simulink model "stage_02"  (R2021b)
settings: Solver=daessc  StartTime=0.0  StopTime=2500  FixedStep=0.001  RelTol=1e-3
values from neighbouring files (symbols this model uses):
  Inom_FC1 = 50    [initParams.m]
  Inom_FC2 = 50    [initParams.m]
  Pnom_FC = 25000    [initParams.m]
  Vnom = 500    [initParams.m]
undefined symbols (not defined in the file or in its folder): Bat, DiscIntNeverNeededParam, Mot
libraries: fl_lib x21, nesl_utility x14, ee_lib x4
settings Model: Creator=gdudgeon  LastModifiedBy=gdudgeon

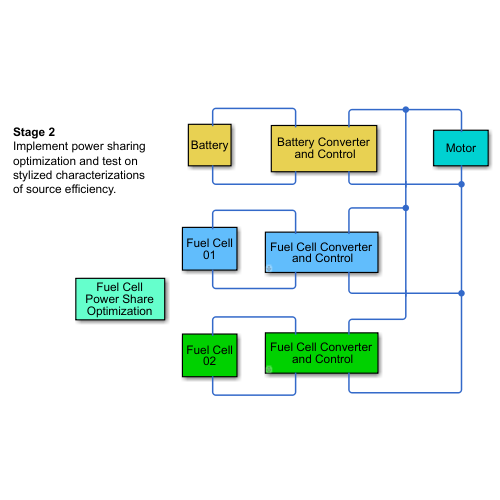
[thumbnail: Simulink's stored preview of the top-level diagram]
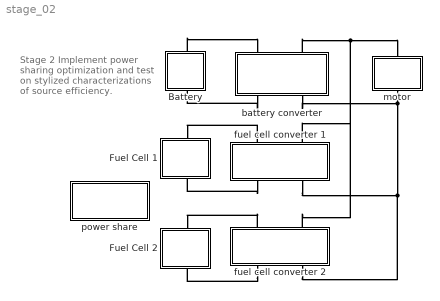
== system stage_02 ==
  note: Stage 2
      | Implement power sharing optimization and test on stylized characterizations of source efficiency.
  Battery : Subsystem
      settings: PortSchema="{\"entries\":[{\"content\":{\"sides\":[{\"content\":{\"connectorIds\":[]},\"type\":\"ConnectorPlacement.EquallySpacedRectSide\",\"uuid\":\"a686e7db-b3c2-4e82-90e1-b07be3e28f3a\"},{\"content\":{\"connectorIds\":[],\"side\":\"RIGHT\"},\"type\":\"ConnectorPlacement.EquallySpacedRectSide\",\"uuid\":\"0e51eb8c-8945-4106-9b2f-04139f0293aa\"},{\"content\":{\"connectorIds\":[\"LConn1\"],\"side\":\"TOP\"},\"type\":\"ConnectorPlacement.EquallySpacedRectSide\",\"uuid\":\"6b60bb75-cfc3-4157-9141-8615eb9e37cb\"},{\"content\":{\"connectorIds\":[\"RConn1\"],\"side\":\"BOTTOM\"},\"type\":\"ConnectorPlacement.EquallySpacedRectSide\",\"uuid\":\"c1a51cb3-7790-499e-bd85-73216263d646\"}]},\"type\":\"ConnectorPlacement.EquallySpacedConnector\",\"uuid\":\"ef7b4de5-6239-4f21-bedd-9a9241ffad20\"}],\"packageUris\":[\"http://schema.mathworks.com/mf0/Connector/R2020b\"],\"version\":\"1.0\"}"
      mask Display: disp('Battery')
  Fuel Cell 1 : Subsystem
      settings: PortSchema="{\"entries\":[{\"content\":{\"sides\":[{\"content\":{\"connectorIds\":[]},\"type\":\"ConnectorPlacement.EquallySpacedRectSide\",\"uuid\":\"a686e7db-b3c2-4e82-90e1-b07be3e28f3a\"},{\"content\":{\"connectorIds\":[],\"side\":\"RIGHT\"},\"type\":\"ConnectorPlacement.EquallySpacedRectSide\",\"uuid\":\"0e51eb8c-8945-4106-9b2f-04139f0293aa\"},{\"content\":{\"connectorIds\":[\"LConn1\"],\"side\":\"TOP\"},\"type\":\"ConnectorPlacement.EquallySpacedRectSide\",\"uuid\":\"6b60bb75-cfc3-4157-9141-8615eb9e37cb\"},{\"content\":{\"connectorIds\":[\"RConn1\"],\"side\":\"BOTTOM\"},\"type\":\"ConnectorPlacement.EquallySpacedRectSide\",\"uuid\":\"6246c242-d76b-4057-8f90-ef1191bb40d6\"}]},\"type\":\"ConnectorPlacement.EquallySpacedConnector\",\"uuid\":\"ef7b4de5-6239-4f21-bedd-9a9241ffad20\"}],\"packageUris\":[\"http://schema.mathworks.com/mf0/Connector/R2020b\"],\"version\":\"1.0\"}"
      mask Display: disp('Fuel Cell\n01')
  Fuel Cell 2 : Subsystem
      settings: PortSchema="{\"entries\":[{\"content\":{\"sides\":[{\"content\":{\"connectorIds\":[]},\"type\":\"ConnectorPlacement.EquallySpacedRectSide\",\"uuid\":\"a686e7db-b3c2-4e82-90e1-b07be3e28f3a\"},{\"content\":{\"connectorIds\":[],\"side\":\"RIGHT\"},\"type\":\"ConnectorPlacement.EquallySpacedRectSide\",\"uuid\":\"0e51eb8c-8945-4106-9b2f-04139f0293aa\"},{\"content\":{\"connectorIds\":[\"LConn1\"],\"side\":\"TOP\"},\"type\":\"ConnectorPlacement.EquallySpacedRectSide\",\"uuid\":\"6b60bb75-cfc3-4157-9141-8615eb9e37cb\"},{\"content\":{\"connectorIds\":[\"RConn1\"],\"side\":\"BOTTOM\"},\"type\":\"ConnectorPlacement.EquallySpacedRectSide\",\"uuid\":\"6246c242-d76b-4057-8f90-ef1191bb40d6\"}]},\"type\":\"ConnectorPlacement.EquallySpacedConnector\",\"uuid\":\"ef7b4de5-6239-4f21-bedd-9a9241ffad20\"}],\"packageUris\":[\"http://schema.mathworks.com/mf0/Connector/R2020b\"],\"version\":\"1.0\"}"
      mask Display: disp('Fuel Cell\n02')
  battery converter : Subsystem
      settings: PortSchema="{\"entries\":[{\"content\":{\"sides\":[{\"content\":{\"connectorIds\":[]},\"type\":\"ConnectorPlacement.EquallySpacedRectSide\",\"uuid\":\"465408c9-80bd-457c-883a-4a132321254b\"},{\"content\":{\"connectorIds\":[],\"side\":\"RIGHT\"},\"type\":\"ConnectorPlacement.EquallySpacedRectSide\",\"uuid\":\"04120ebf-e4ec-443f-a627-4e992580e56f\"},{\"content\":{\"connectorIds\":[\"LConn1\",\"LConn2\"],\"side\":\"TOP\"},\"type\":\"ConnectorPlacement.EquallySpacedRectSide\",\"uuid\":\"0ef2b150-f732-4ac6-bc9b-74fd7e496e19\"},{\"content\":{\"connectorIds\":[\"RConn1\",\"RConn2\"],\"side\":\"BOTTOM\"},\"type\":\"ConnectorPlacement.EquallySpacedRectSide\",\"uuid\":\"3ceaa64c-40e0-49b8-9128-82da92f184b4\"}]},\"type\":\"ConnectorPlacement.EquallySpacedConnector\",\"uuid\":\"70c8e7cc-610c-4e7a-9707-57af70b2f144\"}],\"packageUris\":[\"http://schema.mathworks.com/mf0/Connector/R2020b\"],\"version\":\"1.0\"}"
      mask Display: disp('Battery Converter\n and Control')
  fuel cell converter 1 : Subsystem  mask{Vref=Vnom, Imax=Inom_FC1}
      mask prompts: Vref "Voltage Setpoint (V)"; Imax "Maximum Current (A)"
      settings: PortSchema="{\"entries\":[{\"content\":{\"sides\":[{\"content\":{\"connectorIds\":[]},\"type\":\"ConnectorPlacement.EquallySpacedRectSide\",\"uuid\":\"465408c9-80bd-457c-883a-4a132321254b\"},{\"content\":{\"connectorIds\":[],\"side\":\"RIGHT\"},\"type\":\"ConnectorPlacement.EquallySpacedRectSide\",\"uuid\":\"04120ebf-e4ec-443f-a627-4e992580e56f\"},{\"content\":{\"connectorIds\":[\"LConn1\",\"LConn2\"],\"side\":\"TOP\"},\"type\":\"ConnectorPlacement.EquallySpacedRectSide\",\"uuid\":\"0ef2b150-f732-4ac6-bc9b-74fd7e496e19\"},{\"content\":{\"connectorIds\":[\"RConn1\",\"RConn2\"],\"side\":\"BOTTOM\"},\"type\":\"ConnectorPlacement.EquallySpacedRectSide\",\"uuid\":\"cccf9d02-f6c7-4a15-ab4f-a4dd83d7ce46\"}]},\"type\":\"ConnectorPlacement.EquallySpacedConnector\",\"uuid\":\"70c8e7cc-610c-4e7a-9707-57af70b2f144\"}],\"packageUris\":[\"http://schema.mathworks.com/mf0/Connector/R2020b\"],\"version\":\"1.0\"}"
      mask Display: disp('Fuel Cell Converter\n and Control')
  fuel cell converter 2 : Subsystem  mask{Vref=Vnom, Imax=Inom_FC2}
      mask prompts: Vref "Voltage Setpoint (V)"; Imax "Maximum Current (A)"
      settings: PortSchema="{\"entries\":[{\"content\":{\"sides\":[{\"content\":{\"connectorIds\":[]},\"type\":\"ConnectorPlacement.EquallySpacedRectSide\",\"uuid\":\"465408c9-80bd-457c-883a-4a132321254b\"},{\"content\":{\"connectorIds\":[],\"side\":\"RIGHT\"},\"type\":\"ConnectorPlacement.EquallySpacedRectSide\",\"uuid\":\"04120ebf-e4ec-443f-a627-4e992580e56f\"},{\"content\":{\"connectorIds\":[\"LConn1\",\"LConn2\"],\"side\":\"TOP\"},\"type\":\"ConnectorPlacement.EquallySpacedRectSide\",\"uuid\":\"0ef2b150-f732-4ac6-bc9b-74fd7e496e19\"},{\"content\":{\"connectorIds\":[\"RConn1\",\"RConn2\"],\"side\":\"BOTTOM\"},\"type\":\"ConnectorPlacement.EquallySpacedRectSide\",\"uuid\":\"cccf9d02-f6c7-4a15-ab4f-a4dd83d7ce46\"}]},\"type\":\"ConnectorPlacement.EquallySpacedConnector\",\"uuid\":\"70c8e7cc-610c-4e7a-9707-57af70b2f144\"}],\"packageUris\":[\"http://schema.mathworks.com/mf0/Connector/R2020b\"],\"version\":\"1.0\"}"
      mask Display: disp('Fuel Cell Converter\n and Control')
  motor : Subsystem
      mask Display: disp('Motor')
  power share : Subsystem
      mask Display: disp('Fuel Cell\nPower Share\nOptimization')
  connections:
  motor/RConn1 -- battery converter/RConn2 -- fuel cell converter 2/RConn2 -- fuel cell converter 1/RConn2
  battery converter/LConn2 -- motor/LConn1 -- fuel cell converter 2/LConn2 -- fuel cell converter 1/LConn2
  fuel cell converter 1/LConn1 -- Fuel Cell 1/LConn1
  fuel cell converter 1/RConn1 -- Fuel Cell 1/RConn1
  Battery/LConn1 -- battery converter/LConn1
  battery converter/RConn1 -- Battery/RConn1
  fuel cell converter 2/RConn1 -- Fuel Cell 2/RConn1
  fuel cell converter 2/LConn1 -- Fuel Cell 2/LConn1

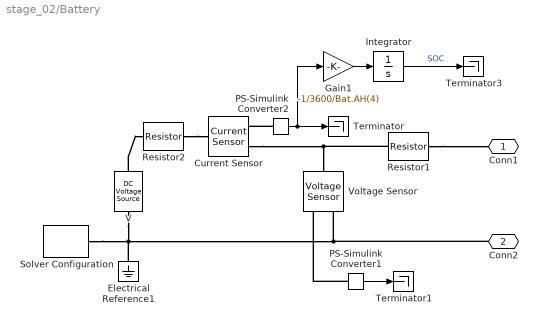
== system stage_02/Battery ==
  Current Sensor : fl_lib/Electrical/Electrical Sensors/Current Sensor
  Electrical Reference1 : fl_lib/Electrical/Electrical Elements/Electrical Reference
  Gain1 : Gain  Gain=-1/3600/Bat.AH(4)
  Integrator : Integrator  InitialCondition=Bat.initSOC
  PS-Simulink Converter1 : nesl_utility/PS-Simulink Converter  PhysicalDomain=network_engine_domain  SubClassName=ps_output  LeftPortType=input  RightPortType=output  PseudoPeriodic=off  Frequencies=[]  Unit=inherit  AffineConversion=off
      settings: SourceProductBaseCode=PW,SS
  PS-Simulink Converter2 : nesl_utility/PS-Simulink Converter  PhysicalDomain=network_engine_domain  SubClassName=ps_output  LeftPortType=input  RightPortType=output  PseudoPeriodic=off  Frequencies=[]  Unit=inherit  AffineConversion=off
      settings: SourceProductBaseCode=PW,SS
  Resistor1 : fl_lib/Electrical/Electrical Elements/Resistor  R=1e-3 Ohm  i_specify=off  i_priority=None  i=0 A  i_nominal_specify=off  i_nominal_unit=A  i_nominal_value=1  v_specify=off  v_priority=None  v=0 V  v_nominal_specify=off  v_nominal_unit=V  v_nominal_value=1
  Resistor2 : fl_lib/Electrical/Electrical Elements/Resistor  R=Bat.R0(4,4) Ohm  i_specify=off  i_priority=None  i=0 A  i_nominal_specify=off  i_nominal_unit=A  i_nominal_value=1  v_specify=off  v_priority=None  v=0 V  v_nominal_specify=off  v_nominal_unit=V  v_nominal_value=1
  Solver Configuration : nesl_utility/Solver Configuration  PhysicalDomain=network_engine_domain  SubClassName=solver  LeftPortType=input  RightPortType=generic  Tones=[]  Harmonics=[]  SimulateNoise=off  Profile=off  UseLocalSampling=off  EnableSwitchedLinearOptims=on  FrequencyDomain=off  UseCCode=off  RelTol=0.001  AbsTol=1e-06  MinStep=1e-09  ToWorkspace=off  RevertToSquareIcSolve=off  NumHomotopyIterations=100  PhasorMode=off  PhasorModeNumHarmonics=1  DoDC=off  ResidualTolerance=1e-09  UseLocalSolver=off  LocalSolverChoice=NE_BACKWARD_EULER_ADVANCER  LocalSolverSampleTime=0.001  DoFixedCost=off  MaxNonlinIter=3  MaxModeIter=2  ComputeImpulses=off  ImpulseIterations=2  LinearAlgebra=auto  EquationFormulation=NE_TIME_EF  DelaysMemoryBudget=1024  AutomaticFiltering=on  FilteringTimeConstant=0.001  PartitionStorageMethod=AS_NEEDED  PartitionMemoryBudget=1024  PartitionMethod=ROBUST
      settings: SourceProductBaseCode=PW,SS
  Terminator : Terminator
  Terminator1 : Terminator
  Terminator3 : Terminator
  V : fl_lib/Electrical/Electrical Sources/DC Voltage Source  v0=Bat.noLoadV(4,4) V
  Voltage Sensor : fl_lib/Electrical/Electrical Sensors/Voltage Sensor
  Conn1 : PMIOPort  Side=Left
  Conn2 : PMIOPort  Port=2  Side=Right
  wires:
  PS-Simulink Converter2/1 -> Gain1/1, Terminator/1
  PS-Simulink Converter1/1 -> Terminator1/1
  Integrator/1 -> Terminator3/1  "SOC"
  Gain1/1 -> Integrator/1
  connections:
  PS-Simulink Converter2/LConn1 -- Current Sensor/RConn1
  Electrical Reference1/LConn1 -- V/RConn1 -- Solver Configuration/RConn1 -- Conn2/RConn1 -- Voltage Sensor/RConn2
  Current Sensor/RConn2 -- Resistor1/LConn1 -- Voltage Sensor/LConn1
  PS-Simulink Converter1/LConn1 -- Voltage Sensor/RConn1
  Resistor1/RConn1 -- Conn1/RConn1
  V/LConn1 -- Resistor2/LConn1
  Resistor2/RConn1 -- Current Sensor/LConn1

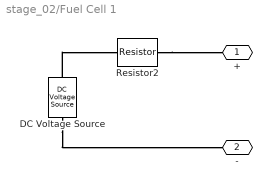
== system stage_02/Fuel Cell 1 ==
  DC Voltage Source : fl_lib/Electrical/Electrical Sources/DC Voltage Source  v0=250 V
  Resistor2 : fl_lib/Electrical/Electrical Elements/Resistor  R=1e-3 Ohm  i_specify=off  i_priority=None  i=0 A  i_nominal_specify=off  i_nominal_unit=A  i_nominal_value=1  v_specify=off  v_priority=None  v=0 V  v_nominal_specify=off  v_nominal_unit=V  v_nominal_value=1
  + : PMIOPort  Side=Left
  - : PMIOPort  Port=2  Side=Right
  connections:
  DC Voltage Source/LConn1 -- Resistor2/LConn1
  Resistor2/RConn1 -- +/RConn1
  DC Voltage Source/RConn1 -- -/RConn1

== system stage_02/Fuel Cell 2 ==
  DC Voltage Source : fl_lib/Electrical/Electrical Sources/DC Voltage Source  v0=250 V
  Resistor2 : fl_lib/Electrical/Electrical Elements/Resistor  R=1e-3 Ohm  i_specify=off  i_priority=None  i=0 A  i_nominal_specify=off  i_nominal_unit=A  i_nominal_value=1  v_specify=off  v_priority=None  v=0 V  v_nominal_specify=off  v_nominal_unit=V  v_nominal_value=1
  + : PMIOPort  Side=Left
  - : PMIOPort  Port=2  Side=Right
  connections:
  DC Voltage Source/RConn1 -- -/RConn1
  Resistor2/RConn1 -- +/RConn1
  DC Voltage Source/LConn1 -- Resistor2/LConn1

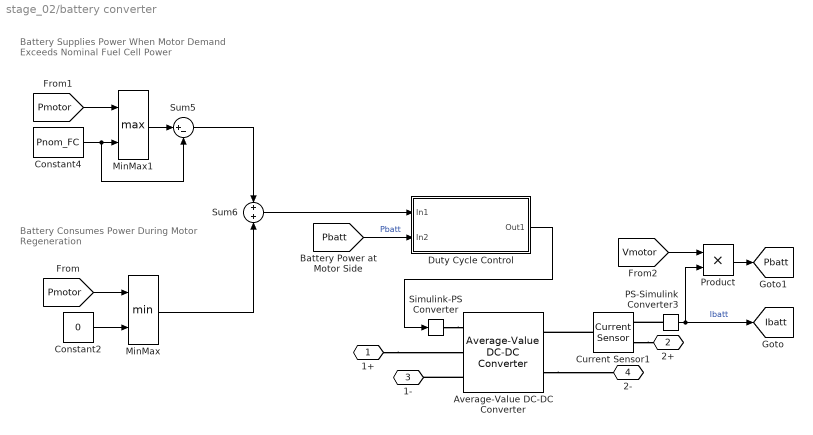
== system stage_02/battery converter ==
  note: Battery Consumes Power
      | During Motor Regeneration
  note: Battery Supplies Power When
      | Motor Demand Exceeds Nominal
      | Fuel Cell Power
  Average-Value DC-DC Converter : ee_lib/Semiconductors & Converters/Converters/Average-Value DC-DC Converter  control_option=ee.enum.converters.controlinput.dutycycle  converter_type=ee.enum.converters.dcdctype.buckboost  efficiency_option=ee.enum.converters.efficiency.constant  efficiency_fixed=100  i_vec=[0, 2, 5] A  efficiency_vec=[90, 95, 98]
      settings: SourceProductBaseCode=PS  InternalSimscapePortConfiguration="{\"Bottom\":[],\"Left\":[{\"id\":\"DutyCycle\",\"label\":\"DutyCycle\",\"type\":\"input\"},{\"id\":\"p1\",\"label\":\"1+\",\"type\":\"foundation.electrical.electrical\"},{\"id\":\"n1\",\"label\":\"1-\",\"type\":\"foundation.electrical.electrical\"}],\"Right\":[{\"id\":\"p2\",\"label\":\"2+\",\"type\":\"foundation.electrical.electrical\"},{\"id\":\"n2\",\"label\":\"2-\",\"type\":\"foundation.electrical.electrical\"}],\"Top\":[]}"
  Constant2 : Constant  Value=0
  Constant4 : Constant  Value=Pnom_FC
  Current Sensor1 : fl_lib/Electrical/Electrical Sensors/Current Sensor
  Duty Cycle Control : Subsystem
      mask Display: disp('Duty-Cycle Control')
  MinMax : MinMax  Inputs=2
  MinMax1 : MinMax  Function=max  Inputs=2
  PS-Simulink Converter3 : nesl_utility/PS-Simulink Converter  PhysicalDomain=network_engine_domain  SubClassName=ps_output  LeftPortType=input  RightPortType=output  PseudoPeriodic=off  Frequencies=[]  Unit=inherit  AffineConversion=off
      settings: SourceProductBaseCode=PW,SS
  Product : Product
  Simulink-PS Converter : nesl_utility/Simulink-PS Converter  PhysicalDomain=network_engine_domain  SubClassName=ps_input  LeftPortType=input  RightPortType=output  PseudoPeriodic=off  Frequencies=[]  NoiseDistribution=none  NoiseParameters=[]  Unit=1  AffineConversion=off  FilteringAndDerivatives=provide  SimscapeFilterOrder=1  InputFilterTimeConstant=0.001  UdotUserProvided=0
      settings: SourceProductBaseCode=PW,SS
  Sum5 : Sum  Inputs=|+-
  Sum6 : Sum
  1+ : PMIOPort  Side=Left
  2+ : PMIOPort  Port=2  Side=Left
  1- : PMIOPort  Port=3  Side=Right
  2- : PMIOPort  Port=4  Side=Right
  tag scope: Ibatt=global, Pbatt=global
  wires:
  Constant4/1 -> Sum5/2, MinMax1/2
  Sum5/1 -> Sum6/1
  MinMax/1 -> Sum6/2
  [Pmotor] -> MinMax1/1
  MinMax1/1 -> Sum5/1
  Constant2/1 -> MinMax/2
  [Pmotor] -> MinMax/1
  PS-Simulink Converter3/1 -> [Ibatt], Product/2  "Ibatt"
  [Pbatt] -> Duty Cycle Control/2(In2)  "Pbatt"
  Duty Cycle Control/1(Out1) -> Simulink-PS Converter/1
  Sum6/1 -> Duty Cycle Control/1(In1)
  [Vmotor] -> Product/1
  Product/1 -> [Pbatt]
  connections:
  PS-Simulink Converter3/LConn1 -- Current Sensor1/RConn1
  Average-Value DC-DC Converter/RConn2 -- 2-/RConn1
  Current Sensor1/LConn1 -- Average-Value DC-DC Converter/RConn1
  Average-Value DC-DC Converter/LConn3 -- 1-/RConn1
  1+/RConn1 -- Average-Value DC-DC Converter/LConn2
  Simulink-PS Converter/RConn1 -- Average-Value DC-DC Converter/LConn1
  Current Sensor1/RConn2 -- 2+/RConn1

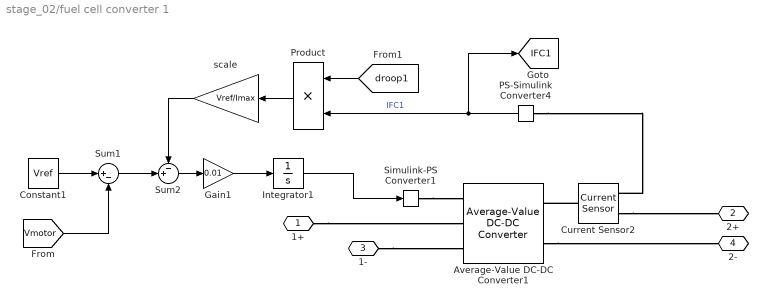
== system stage_02/fuel cell converter 1 ==
  Average-Value DC-DC Converter1 : ee_lib/Semiconductors & Converters/Converters/Average-Value DC-DC Converter  control_option=ee.enum.converters.controlinput.dutycycle  converter_type=ee.enum.converters.dcdctype.buckboost  efficiency_option=ee.enum.converters.efficiency.constant  efficiency_fixed=100  i_vec=[0, 2, 5] A  efficiency_vec=[90, 95, 98]
      settings: SourceProductBaseCode=PS  InternalSimscapePortConfiguration="{\"Bottom\":[],\"Left\":[{\"id\":\"DutyCycle\",\"label\":\"DutyCycle\",\"type\":\"input\"},{\"id\":\"p1\",\"label\":\"1+\",\"type\":\"foundation.electrical.electrical\"},{\"id\":\"n1\",\"label\":\"1-\",\"type\":\"foundation.electrical.electrical\"}],\"Right\":[{\"id\":\"p2\",\"label\":\"2+\",\"type\":\"foundation.electrical.electrical\"},{\"id\":\"n2\",\"label\":\"2-\",\"type\":\"foundation.electrical.electrical\"}],\"Top\":[]}"
  Constant1 : Constant  Value=Vref
  Current Sensor2 : fl_lib/Electrical/Electrical Sensors/Current Sensor
  Gain1 : Gain  Gain=0.01
  Integrator1 : Integrator  InitialCondition=0.5
  PS-Simulink Converter4 : nesl_utility/PS-Simulink Converter  PhysicalDomain=network_engine_domain  SubClassName=ps_output  LeftPortType=input  RightPortType=output  PseudoPeriodic=off  Frequencies=[]  Unit=inherit  AffineConversion=off
      settings: SourceProductBaseCode=PW,SS
  Product : Product
  Simulink-PS Converter1 : nesl_utility/Simulink-PS Converter  PhysicalDomain=network_engine_domain  SubClassName=ps_input  LeftPortType=input  RightPortType=output  PseudoPeriodic=off  Frequencies=[]  NoiseDistribution=none  NoiseParameters=[]  Unit=1  AffineConversion=off  FilteringAndDerivatives=provide  SimscapeFilterOrder=1  InputFilterTimeConstant=0.001  UdotUserProvided=0
      settings: SourceProductBaseCode=PW,SS
  Sum1 : Sum  Inputs=|+-
  Sum2 : Sum  Inputs=-+|
  scale : Gain  Gain=Vref/Imax
  1+ : PMIOPort  Side=Left
  2+ : PMIOPort  Port=2  Side=Left
  1- : PMIOPort  Port=3  Side=Right
  2- : PMIOPort  Port=4  Side=Right
  tag scope: IFC1=global
  wires:
  Sum2/1 -> Gain1/1
  Sum1/1 -> Sum2/2
  Constant1/1 -> Sum1/1
  scale/1 -> Sum2/1
  PS-Simulink Converter4/1 -> Product/2, [IFC1]  "IFC1"
  Integrator1/1 -> Simulink-PS Converter1/1
  Gain1/1 -> Integrator1/1
  [Vmotor] -> Sum1/2
  [droop1] -> Product/1
  Product/1 -> scale/1
  connections:
  Current Sensor2/RConn2 -- 2+/RConn1
  Current Sensor2/LConn1 -- Average-Value DC-DC Converter1/RConn1
  PS-Simulink Converter4/LConn1 -- Current Sensor2/RConn1
  Simulink-PS Converter1/RConn1 -- Average-Value DC-DC Converter1/LConn1
  1-/RConn1 -- Average-Value DC-DC Converter1/LConn3
  Average-Value DC-DC Converter1/RConn2 -- 2-/RConn1
  1+/RConn1 -- Average-Value DC-DC Converter1/LConn2

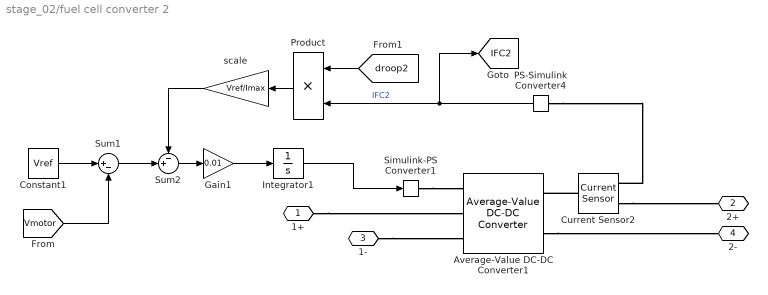
== system stage_02/fuel cell converter 2 ==
  Average-Value DC-DC Converter1 : ee_lib/Semiconductors & Converters/Converters/Average-Value DC-DC Converter  control_option=ee.enum.converters.controlinput.dutycycle  converter_type=ee.enum.converters.dcdctype.buckboost  efficiency_option=ee.enum.converters.efficiency.constant  efficiency_fixed=100  i_vec=[0, 2, 5] A  efficiency_vec=[90, 95, 98]
      settings: SourceProductBaseCode=PS  InternalSimscapePortConfiguration="{\"Bottom\":[],\"Left\":[{\"id\":\"DutyCycle\",\"label\":\"DutyCycle\",\"type\":\"input\"},{\"id\":\"p1\",\"label\":\"1+\",\"type\":\"foundation.electrical.electrical\"},{\"id\":\"n1\",\"label\":\"1-\",\"type\":\"foundation.electrical.electrical\"}],\"Right\":[{\"id\":\"p2\",\"label\":\"2+\",\"type\":\"foundation.electrical.electrical\"},{\"id\":\"n2\",\"label\":\"2-\",\"type\":\"foundation.electrical.electrical\"}],\"Top\":[]}"
  Constant1 : Constant  Value=Vref
  Current Sensor2 : fl_lib/Electrical/Electrical Sensors/Current Sensor
  Gain1 : Gain  Gain=0.01
  Integrator1 : Integrator  InitialCondition=0.5
  PS-Simulink Converter4 : nesl_utility/PS-Simulink Converter  PhysicalDomain=network_engine_domain  SubClassName=ps_output  LeftPortType=input  RightPortType=output  PseudoPeriodic=off  Frequencies=[]  Unit=inherit  AffineConversion=off
      settings: SourceProductBaseCode=PW,SS
  Product : Product
  Simulink-PS Converter1 : nesl_utility/Simulink-PS Converter  PhysicalDomain=network_engine_domain  SubClassName=ps_input  LeftPortType=input  RightPortType=output  PseudoPeriodic=off  Frequencies=[]  NoiseDistribution=none  NoiseParameters=[]  Unit=1  AffineConversion=off  FilteringAndDerivatives=provide  SimscapeFilterOrder=1  InputFilterTimeConstant=0.001  UdotUserProvided=0
      settings: SourceProductBaseCode=PW,SS
  Sum1 : Sum  Inputs=|+-
  Sum2 : Sum  Inputs=-+|
  scale : Gain  Gain=Vref/Imax
  1+ : PMIOPort  Side=Left
  2+ : PMIOPort  Port=2  Side=Left
  1- : PMIOPort  Port=3  Side=Right
  2- : PMIOPort  Port=4  Side=Right
  tag scope: IFC2=global
  wires:
  [Vmotor] -> Sum1/2
  Gain1/1 -> Integrator1/1
  Integrator1/1 -> Simulink-PS Converter1/1
  PS-Simulink Converter4/1 -> Product/2, [IFC2]  "IFC2"
  scale/1 -> Sum2/1
  Constant1/1 -> Sum1/1
  Sum1/1 -> Sum2/2
  Sum2/1 -> Gain1/1
  Product/1 -> scale/1
  [droop2] -> Product/1
  connections:
  1+/RConn1 -- Average-Value DC-DC Converter1/LConn2
  Average-Value DC-DC Converter1/RConn2 -- 2-/RConn1
  1-/RConn1 -- Average-Value DC-DC Converter1/LConn3
  Simulink-PS Converter1/RConn1 -- Average-Value DC-DC Converter1/LConn1
  PS-Simulink Converter4/LConn1 -- Current Sensor2/RConn1
  Current Sensor2/LConn1 -- Average-Value DC-DC Converter1/RConn1
  Current Sensor2/RConn2 -- 2+/RConn1

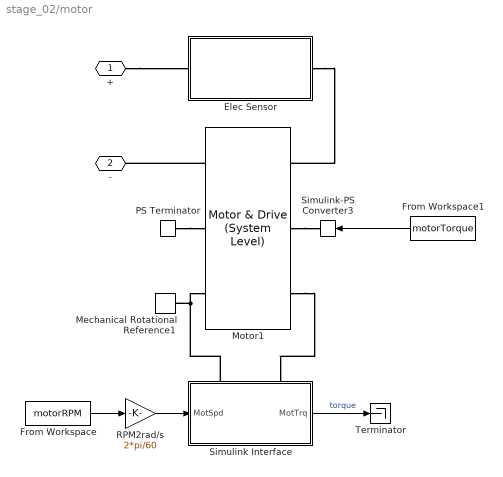
== system stage_02/motor ==
  Elec Sensor : Subsystem
  From Workspace : FromWorkspace  VariableName=motorRPM
  From Workspace1 : FromWorkspace  VariableName=motorTorque
  Mechanical Rotational Reference1 : fl_lib/Mechanical/Rotational Elements/Mechanical Rotational Reference
  Motor1 : ee_lib/Electromechanical/Motor & Drive (System Level)  torque_speed_param=ee.enum.electromech.envelope.tabulated  overtorque_param=ee.enum.electromech.overtorque.no  T_t=Mot.maxT N*m  T_t_intermittent=[.36, .32, .28, 0] N*m  w_t=Mot.w_eff_bp rpm  torque_max=0.1 N*m  power_max=30 W  torque_max_intermittent=0.4 N*m  power_max_intermittent=120 W  time_overtorque=30 s  time_recover=60 s  Tc=Mot.Tc_Mot s  losses_param=3  eff=100  w_eff=3750 rpm  T_eff=0.08 N*m  Piron=0 W  Pbase=0 W  w_eff_vec=Mot.w_eff_bp rpm  T_eff_vec=Mot.T_eff_bp N*m  v_eff_vec=[100, 250, 400] V  losses_mat=[1.49, 1.67, 2.21, 3.1; .42, .69, 1.14, 2.03; .06, .24, .78, 1.68; .42, .69, 1.14, 2.03; 1.49, 1.67, 2.21, 3.1] W  efficiency_mat=Mot.efficiency_table  losses_mat_3D=ones(5, 4, 3) W  efficiency_mat_3D=95 * ones(5, 4, 3)  Res=Mot.supplyRes Ohm  enable_fault=simscape.enum.onoff.off  fault_condition=1  fault_threshold=0.5  J=Mot.inertia kg*m^2  lam=Mot.damping N*m/(rad/s)  speed0=0 rpm  faulted_specify=off  faulted_priority=None  faulted=0  faulted_nominal_specify=off  faulted_nominal_unit=1  faulted_nominal_value=1  torqueLimitContinuous_specify=off  torqueLimitContinuous_priority=None  torqueLimitContinuous=0 N*m  torqueLimitContinuous_nominal_specify=off  torqueLimitContinuous_nominal_unit=N*m  torqueLimitContinuous_nominal_value=1  alpha=3.93e-3 1/K  Tmeas=25 degC  Tmeas2=125 degC  losses_mat_T2=[1.49, 1.74, 2.49, 3.74; .42, .67, 1.42, 2.67; .06, .31, 1.06, 2.31; .42, .67, 1.42, 2.67; 1.49, 1.74, 2.49, 3.74] W  efficiency_mat_T2=[95, 95, 95, 95; 95, 95, 95, 95; 95, 95, 95, 95; 95, 95, 95, 95; 95, 95, 95, 95]  losses_mat_3D_T2=ones(5, 4, 3) W  efficiency_mat_3D_T2=95 * ones(5, 4, 3)  thermal_mass=100 J/K  initial_temperature=25 degC
      settings: SourceProductBaseCode=PS
  PS Terminator : fl_lib/Physical Signals/Sinks/PS Terminator
  RPM2rad/s : Gain  Gain=2*pi/60
  Simulink Interface : Subsystem
      settings: PortSchema="{\"entries\":[{\"content\":{\"sides\":[{\"content\":{\"connectorIds\":[\"In1\"]},\"type\":\"ConnectorPlacement.EquallySpacedRectSide\",\"uuid\":\"bf4125d2-d804-43ee-b309-19af55b24a20\"},{\"content\":{\"connectorIds\":[\"Out1\"],\"side\":\"RIGHT\"},\"type\":\"ConnectorPlacement.EquallySpacedRectSide\",\"uuid\":\"b387e632-ddea-4493-9ae8-5e997efec9a6\"},{\"content\":{\"connectorIds\":[\"LConn1\",\"LConn2\"],\"side\":\"TOP\"},\"type\":\"ConnectorPlacement.EquallySpacedRectSide\",\"uuid\":\"41fd5ea6-0488-466e-8be0-697a42498d14\"}]},\"type\":\"ConnectorPlacement.EquallySpacedConnector\",\"uuid\":\"25cf6a75-933f-4ef5-8c77-b93f7c2ffe1f\"}],\"packageUris\":[\"http://schema.mathworks.com/mf0/Connector/R2020b\"],\"version\":\"1.0\"}"
  Simulink-PS Converter3 : nesl_utility/Simulink-PS Converter  PhysicalDomain=network_engine_domain  SubClassName=ps_input  LeftPortType=input  RightPortType=output  PseudoPeriodic=off  Frequencies=[]  NoiseDistribution=none  NoiseParameters=[]  Unit=N*m  AffineConversion=off  FilteringAndDerivatives=provide  SimscapeFilterOrder=1  InputFilterTimeConstant=0.001  UdotUserProvided=0
      settings: SourceProductBaseCode=PW,SS
  Terminator : Terminator
  + : PMIOPort  Side=Left
  - : PMIOPort  Port=2  Side=Right
  wires:
  RPM2rad/s/1 -> Simulink Interface/1(MotSpd)
  Simulink Interface/1(MotTrq) -> Terminator/1  "torque"
  From Workspace/1 -> RPM2rad/s/1
  From Workspace1/1 -> Simulink-PS Converter3/1
  connections:
  Mechanical Rotational Reference1/LConn1 -- Motor1/RConn3 -- Simulink Interface/LConn1
  PS Terminator/LConn1 -- Motor1/RConn2
  Elec Sensor/RConn1 -- Motor1/LConn1
  Motor1/LConn2 -- Simulink-PS Converter3/RConn1
  Motor1/LConn3 -- Simulink Interface/LConn2
  Motor1/RConn1 -- -/RConn1
  +/RConn1 -- Elec Sensor/LConn1

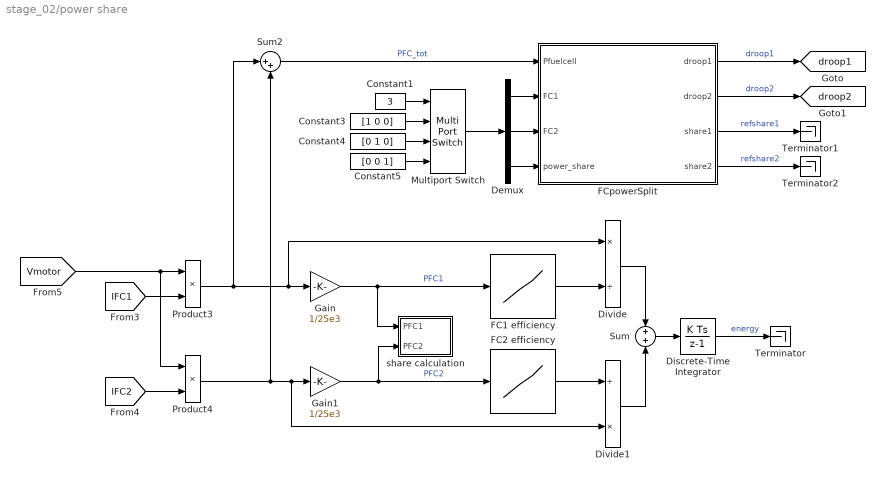
== system stage_02/power share ==
  Constant1 : Constant  Value=3
  Constant3 : Constant  Value=[1 0 0]
  Constant4 : Constant  Value=[0 1 0]
  Constant5 : Constant  Value=[0 0 1]
  Demux : Demux  Outputs=3
  Discrete-Time Integrator : DiscreteIntegrator  SampleTime=0.01  ICPrevOutput=DiscIntNeverNeededParam  ICPrevScaledInput=DiscIntNeverNeededParam
  Divide : Product  Inputs=*/
  Divide1 : Product  Inputs=/*
  FC1 efficiency : Lookup_n-D  NumberOfTableDimensions=1  BreakpointsForDimension1=[0 1]  Table=[0.8 0.2]  InternalRulePriority=Speed  RndMeth=Simplest  InputSameDT=on
  FC2 efficiency : Lookup_n-D  NumberOfTableDimensions=1  BreakpointsForDimension1=[0 1]  Table=[0.6 0.4]  InternalRulePriority=Speed  RndMeth=Simplest  InputSameDT=on
  FCpowerSplit : MATLAB Function  TreatAsAtomicUnit=on  SystemSampleTime=Tanim  mask(Fuel Cell Power Share){Tanim=1}
      mask prompts: Tanim "Update Rate [s]"
      mask help: This block optimizes the power share of two fuel cell units in parallel based on efficiency curves.
  Gain : Gain  Gain=1/25e3
  Gain1 : Gain  Gain=1/25e3
  Multiport Switch : MultiPortSwitch
  Product3 : Product
  Product4 : Product
  Sum : Sum
  Sum2 : Sum  Inputs=|++
  Terminator : Terminator
  Terminator1 : Terminator
  Terminator2 : Terminator
  share calculation : Subsystem
  tag scope: droop1=global, droop2=global
  wires:
  FCpowerSplit/2(droop2) -> [droop2]  "droop2"
  FCpowerSplit/1(droop1) -> [droop1]  "droop1"
  Gain/1 -> share calculation/1(PFC1), FC1 efficiency/1  "PFC1"
  Gain1/1 -> FC2 efficiency/1, share calculation/2(PFC2)  "PFC2"
  Divide/1 -> Sum/1
  Divide1/1 -> Sum/2
  Sum/1 -> Discrete-Time Integrator/1
  Discrete-Time Integrator/1 -> Terminator/1  "energy"
  Sum2/1 -> FCpowerSplit/1(Pfuelcell)  "PFC_tot"
  Product3/1 -> Sum2/1, Divide/1, Gain/1
  Product4/1 -> Gain1/1, Divide1/2, Sum2/2
  FC1 efficiency/1 -> Divide/2
  FC2 efficiency/1 -> Divide1/1
  FCpowerSplit/3(share1) -> Terminator1/1  "refshare1"
  FCpowerSplit/4(share2) -> Terminator2/1  "refshare2"
  Multiport Switch/1 -> Demux/1
  Constant1/1 -> Multiport Switch/1
  Constant4/1 -> Multiport Switch/3
  Constant5/1 -> Multiport Switch/4
  Constant3/1 -> Multiport Switch/2
  Demux/2 -> FCpowerSplit/3(FC2)
  Demux/1 -> FCpowerSplit/2(FC1)
  Demux/3 -> FCpowerSplit/4(power_share)
  [Vmotor] -> Product4/1, Product3/1
  [IFC2] -> Product4/2
  [IFC1] -> Product3/2

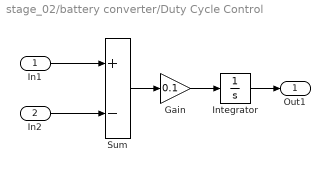
== system stage_02/battery converter/Duty Cycle Control ==
  In1 : Inport
  In2 : Inport  Port=2
  Gain : Gain  Gain=0.1
  Integrator : Integrator  InitialCondition=0.5
  Sum : Sum  Inputs=+-
  Out1 : Outport
  wires:
  Gain/1 -> Integrator/1
  Integrator/1 -> Out1/1
  Sum/1 -> Gain/1
  In1/1 -> Sum/1
  In2/1 -> Sum/2

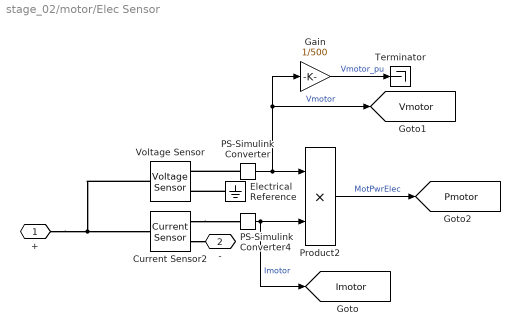
== system stage_02/motor/Elec Sensor ==
  Current Sensor2 : fl_lib/Electrical/Electrical Sensors/Current Sensor
  Electrical Reference : fl_lib/Electrical/Electrical Elements/Electrical Reference
  Gain : Gain  Gain=1/500
  PS-Simulink Converter : nesl_utility/PS-Simulink Converter  PhysicalDomain=network_engine_domain  SubClassName=ps_output  LeftPortType=input  RightPortType=output  PseudoPeriodic=off  Frequencies=[]  Unit=inherit  AffineConversion=off
      settings: SourceProductBaseCode=PW,SS
  PS-Simulink Converter4 : nesl_utility/PS-Simulink Converter  PhysicalDomain=network_engine_domain  SubClassName=ps_output  LeftPortType=input  RightPortType=output  PseudoPeriodic=off  Frequencies=[]  Unit=1  AffineConversion=off
      settings: SourceProductBaseCode=PW,SS
  Product2 : Product
  Terminator : Terminator
  Voltage Sensor : fl_lib/Electrical/Electrical Sensors/Voltage Sensor
  + : PMIOPort  Side=Left
  - : PMIOPort  Port=2  Side=Right
  tag scope: Imotor=global, Pmotor=global, Vmotor=global
  wires:
  PS-Simulink Converter4/1 -> Product2/2, [Imotor]  "Imotor"
  Product2/1 -> [Pmotor]  "MotPwrElec"
  PS-Simulink Converter/1 -> Gain/1, [Vmotor], Product2/1  "Vmotor"
  Gain/1 -> Terminator/1  "Vmotor_pu"
  connections:
  Current Sensor2/RConn1 -- PS-Simulink Converter4/LConn1
  Current Sensor2/RConn2 -- -/RConn1
  +/RConn1 -- Voltage Sensor/LConn1 -- Current Sensor2/LConn1
  Electrical Reference/LConn1 -- Voltage Sensor/RConn2
  PS-Simulink Converter/LConn1 -- Voltage Sensor/RConn1

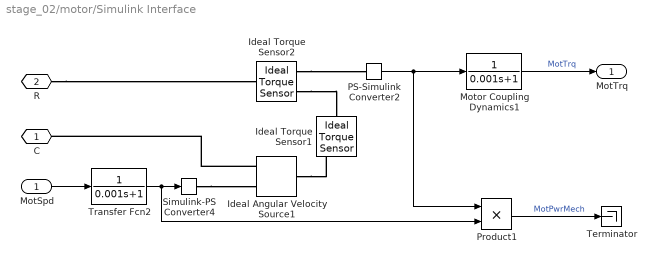
== system stage_02/motor/Simulink Interface ==
  MotSpd : Inport
  Ideal Angular Velocity Source1 : fl_lib/Mechanical/Mechanical Sources/Ideal Angular Velocity Source
  Ideal Torque Sensor1 : fl_lib/Mechanical/Mechanical Sensors/Ideal Torque Sensor
  Ideal Torque Sensor2 : fl_lib/Mechanical/Mechanical Sensors/Ideal Torque Sensor
  Motor Coupling Dynamics1 : TransferFcn  Denominator=[0.001 1]
  PS-Simulink Converter2 : nesl_utility/PS-Simulink Converter  PhysicalDomain=network_engine_domain  SubClassName=ps_output  LeftPortType=input  RightPortType=output  PseudoPeriodic=off  Frequencies=[]  Unit=1  AffineConversion=off
      settings: SourceProductBaseCode=PW,SS
  Product1 : Product
  Simulink-PS Converter4 : nesl_utility/Simulink-PS Converter  PhysicalDomain=network_engine_domain  SubClassName=ps_input  LeftPortType=input  RightPortType=output  PseudoPeriodic=off  Frequencies=[]  NoiseDistribution=none  NoiseParameters=[]  Unit=rad/s  AffineConversion=off  FilteringAndDerivatives=filter  SimscapeFilterOrder=1  InputFilterTimeConstant=0.001  UdotUserProvided=0
      settings: SourceProductBaseCode=PW,SS
  Terminator : Terminator
  Transfer Fcn2 : TransferFcn  Denominator=[0.001 1]
  C : PMIOPort  Side=Left
  R : PMIOPort  Port=2  Side=Left
  MotTrq : Outport
  wires:
  Motor Coupling Dynamics1/1 -> MotTrq/1  "MotTrq"
  MotSpd/1 -> Transfer Fcn2/1
  PS-Simulink Converter2/1 -> Product1/1, Motor Coupling Dynamics1/1
  Transfer Fcn2/1 -> Product1/2, Simulink-PS Converter4/1
  Product1/1 -> Terminator/1  "MotPwrMech"
  connections:
  Ideal Torque Sensor2/RConn2 -- PS-Simulink Converter2/LConn1
  Ideal Angular Velocity Source1/LConn1 -- Ideal Torque Sensor1/RConn1
  Simulink-PS Converter4/RConn1 -- Ideal Angular Velocity Source1/RConn1
  Ideal Torque Sensor2/RConn1 -- Ideal Torque Sensor1/LConn1
  Ideal Angular Velocity Source1/RConn2 -- C/RConn1
  R/RConn1 -- Ideal Torque Sensor2/LConn1

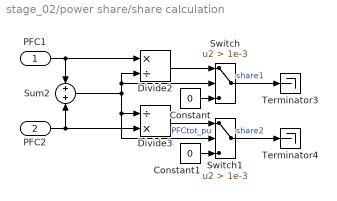
== system stage_02/power share/share calculation ==
  PFC1 : Inport
  PFC2 : Inport  Port=2
  Constant : Constant  Value=0
  Constant1 : Constant  Value=0
  Divide2 : Product  Inputs=*/
  Divide3 : Product  Inputs=/*
  Sum2 : Sum
  Switch : Switch  Criteria=u2 > Threshold  Threshold=1e-3
  Switch1 : Switch  Criteria=u2 > Threshold  Threshold=1e-3
  Terminator3 : Terminator
  Terminator4 : Terminator
  wires:
  Sum2/1 -> Divide2/2, Switch/2, Divide3/1, Switch1/2  "PFCtot_pu"
  Divide3/1 -> Switch1/1
  Switch/1 -> Terminator3/1  "share1"
  Switch1/1 -> Terminator4/1  "share2"
  PFC2/1 -> Sum2/2, Divide3/2
  Divide2/1 -> Switch/1
  PFC1/1 -> Sum2/1, Divide2/1
  Constant1/1 -> Switch1/3
  Constant/1 -> Switch/3

== matlab function stage_02/power share/FCpowerSplit ==
  data: Pfuelcell input; droop1 output; droop2 output; FC1 input; FC2 input; power_share input; share1 output; share2 output
function [droop1,droop2,share1,share2] = FCpowerSplitStage2(Pfuelcell,FC1,FC2,power_share)

coder.extrinsic('powerShare2UnitsStage2')

x = [1 1];

xx = Pfuelcell/25000;

x = powerShare2UnitsStage2(xx);

% default power share is 50-50 with 5% droop

droop1 = 0.05;
droop2 = 0.05;

% optimized power share

if x(1)>1e-3 || x(2)>1e-3
    share1 = x(1)/(sum(x));
    share2 = x(2)/(sum(x));
else
    share1 = 0;
    share2 = 0;
end


% modify droop values based on power share

if Pfuelcell > 500 && power_share

    if x(1) >= x(2)

        droop1 = 0.05;
        droop2 = min(10,droop1*x(1)/x(2));

    else

        droop2 = 0.05;
        droop1 = min(10,droop2*x(2)/x(1));

    end

elseif FC1

    droop1 = 0;
    droop2 = 0.05;
    share1 = 1;
    share2 = 0;

elseif FC2

    droop1 = 0.05;
    droop2 = 0 ;
    share1 = 0;
    share2 = 1;
else

    droop1 = 0.05;
    droop2 = 0.05;

end

end
